simulink model "FlFltCtl_Ht"  (R2016b)
settings: configuration reference "CodeGenConfigSet" (kept outside this file)
values from neighbouring files (symbols this model uses):
  FlFltCtl_nHtThres_C = Calibration.Parameter    [init_FlFltCtl_Ht.m]    (also in init_FlFltCtl_Ht_SIL.m = Simulink.Parameter)
  FlFltCtl_SwtSigSel_C = Calibration.Parameter    [init_FlFltCtl_Ht.m]    (also in init_FlFltCtl_Ht_SIL.m = Simulink.Parameter)
  FlFltCtl_tHysHi_C = Calibration.Parameter    [init_FlFltCtl_Ht.m]    (also in init_FlFltCtl_Ht_SIL.m = Simulink.Parameter)
  FlFltCtl_tHysLo_C = Calibration.Parameter    [init_FlFltCtl_Ht.m]    (also in init_FlFltCtl_Ht_SIL.m = Simulink.Parameter)
undefined symbols (not defined in the file or in its folder): EngState_conv
libraries: CXLib x1
settings Model: Creator=liutao  LastModifiedBy=liutao
settings ConfigSetRef: SourceLocation=Base Workspace

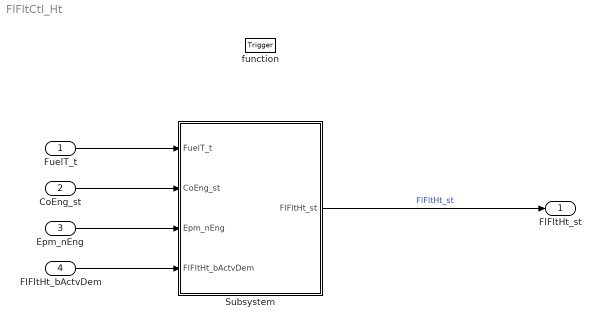
== system FlFltCtl_Ht ==
  FuelT_t : Inport  Tag=deg  Description=Temperature of fuel  OutMin=-50  OutMax=150  OutDataTypeStr=Temp_deg
  CoEng_st : Inport  Description=Engine coordinator state  Port=2  OutDataTypeStr=Enum: EngState_conv
  Epm_nEng : Inport  Tag=rpm  Description=Engine speed  Port=3  OutMin=0  OutMax=6000  OutDataTypeStr=EngSpeed_rpm
  FlFltHt_bActvDem : Inport  Description=|  Port=4  OutMin=0  OutMax=1  OutDataTypeStr=boolean
      | Status of Fuel Filter Heating Digital output received
      | over CAN
  function : TriggerPort  TriggerType=function-call  VariantControl=Variant
  Subsystem : Subsystem
  FlFltHt_st : Outport  Description=Status of Fuel Filter Heating Digital output  OutMin=0  OutMax=1  OutDataTypeStr=boolean
  wires:
  Subsystem/1(FlFltHt_st) -> FlFltHt_st/1  "FlFltHt_st"
  FuelT_t/1 -> Subsystem/1(FuelT_t)
  CoEng_st/1 -> Subsystem/2(CoEng_st)
  FlFltHt_bActvDem/1 -> Subsystem/4(FlFltHt_bActvDem)
  Epm_nEng/1 -> Subsystem/3(Epm_nEng)

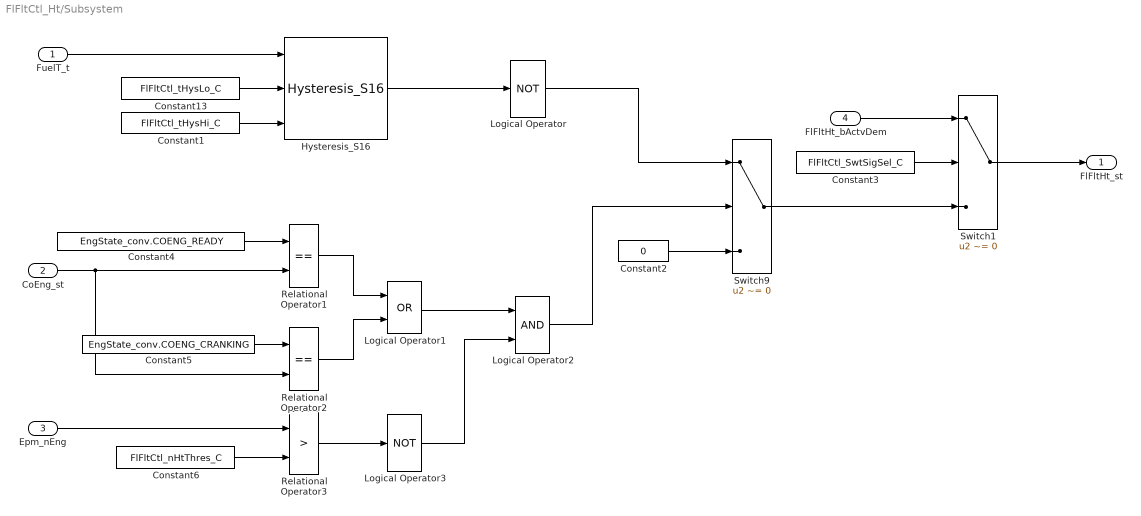
== system FlFltCtl_Ht/Subsystem ==
  FuelT_t : Inport  Tag=deg  Description=Temperature of fuel
  CoEng_st : Inport  Description=Engine coordinator state  Port=2
  Epm_nEng : Inport  Tag=rpm  Description=Engine speed  Port=3
  FlFltHt_bActvDem : Inport  Description=|  Port=4
      | Status of Fuel Filter Heating Digital output received
      | over CAN
  Constant1 : Constant  Value=FlFltCtl_tHysHi_C  SampleTime=-1
  Constant13 : Constant  Value=FlFltCtl_tHysLo_C  SampleTime=-1
  Constant2 : Constant  Value=0  OutDataTypeStr=boolean  SampleTime=-1
  Constant3 : Constant  Value=FlFltCtl_SwtSigSel_C  SampleTime=-1
  Constant4 : Constant  Value=EngState_conv.COENG_READY  OutDataTypeStr=Enum:EngState_conv  SampleTime=-1
  Constant5 : Constant  Value=EngState_conv.COENG_CRANKING  OutDataTypeStr=Enum:EngState_conv  SampleTime=-1
  Constant6 : Constant  Value=FlFltCtl_nHtThres_C  SampleTime=-1
  Hysteresis_S16 : CXLib/Hysteresis_S16
  Logical Operator : Logic  Operator=NOT  Inputs=1  AllPortsSameDT=off  OutDataTypeStr=boolean
  Logical Operator1 : Logic  Operator=OR  OutDataTypeStr=boolean
  Logical Operator2 : Logic  OutDataTypeStr=boolean
  Logical Operator3 : Logic  Operator=NOT  Inputs=1  AllPortsSameDT=off  OutDataTypeStr=boolean
  Relational Operator1 : RelationalOperator  Operator===  OutDataTypeStr=boolean  RndMeth=Nearest  InputSameDT=on
  Relational Operator2 : RelationalOperator  Operator===  OutDataTypeStr=boolean  RndMeth=Nearest  InputSameDT=on
  Relational Operator3 : RelationalOperator  Operator=>  OutDataTypeStr=boolean  RndMeth=Nearest  InputSameDT=on
  Switch1 : Switch  Criteria=u2 ~= 0  InputSameDT=on
  Switch9 : Switch  Criteria=u2 ~= 0  InputSameDT=on
  FlFltHt_st : Outport  Description=Status of Fuel Filter Heating Digital output  OutMin=0  OutMax=1
  wires:
  FuelT_t/1 -> Hysteresis_S16/1
  Constant13/1 -> Hysteresis_S16/2
  Constant1/1 -> Hysteresis_S16/3
  Hysteresis_S16/1 -> Logical Operator/1
  Logical Operator/1 -> Switch9/1
  Constant2/1 -> Switch9/3
  Switch1/1 -> FlFltHt_st/1
  Constant3/1 -> Switch1/2
  Switch9/1 -> Switch1/3
  Constant4/1 -> Relational Operator1/1
  CoEng_st/1 -> Relational Operator2/2, Relational Operator1/2
  Constant5/1 -> Relational Operator2/1
  Relational Operator1/1 -> Logical Operator1/1
  Relational Operator2/1 -> Logical Operator1/2
  Logical Operator1/1 -> Logical Operator2/1
  Constant6/1 -> Relational Operator3/2
  Epm_nEng/1 -> Relational Operator3/1
  Logical Operator2/1 -> Switch9/2
  FlFltHt_bActvDem/1 -> Switch1/1
  Relational Operator3/1 -> Logical Operator3/1
  Logical Operator3/1 -> Logical Operator2/2
